simulink subsystem "directFFcontroller"  (R2021a)
settings: Solver=VariableStepAuto  StartTime=0.0  StopTime=10.0  RelTol=1e-3
settings Model: Creator=chukh  LastModifiedBy=chukh

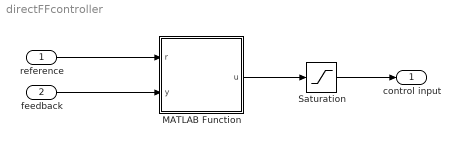
== system directFFcontroller ==
  reference : Inport
  feedback : Inport  Port=2
  MATLAB Function : MATLAB Function  TreatAsAtomicUnit=on
  Saturation : Saturate  UpperLimit=1.0  LowerLimit=0.0
  control input : Outport
  wires:
  reference/1 -> MATLAB Function/1(r)
  Saturation/1 -> control input/1
  MATLAB Function/1(u) -> Saturation/1
  feedback/1 -> MATLAB Function/2(y)

== matlab function directFFcontroller/MATLAB Function ==
  data: r input; u output; y input
function u = fcn(r,y)

u = double(r);
